simulink model "lab_single_phse_inv"  (R2020a)
settings: Solver=VariableStepAuto  StartTime=0.0  StopTime=0.1  RelTol=1e-3
libraries: powerlib x9, simulink x1
settings Model: Creator=Manish  LastModifiedBy=Manish
settings DataIOCC: ReturnWorkspaceOutputs=off

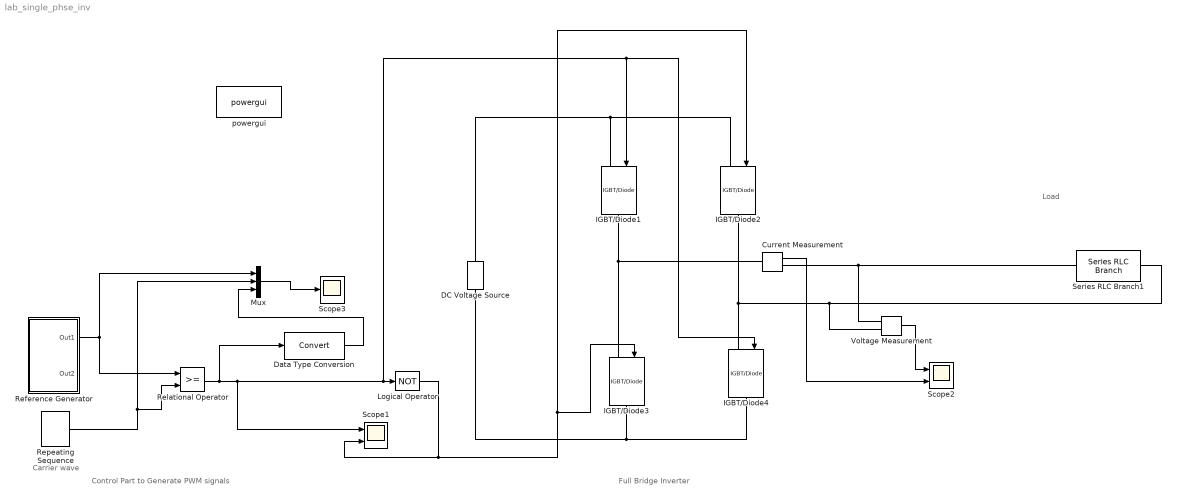
== system lab_single_phse_inv ==
  note: Full Bridge Inverter
  note: Load
  note: Control Part to
      | Generate PWM signals
  note: Carrier wave
  Current Measurement : powerlib/Measurements/Current Measurement  PhasorSimulation=off  OutputType=Complex  PSBequivalent=0
  DC Voltage Source : powerlib/Electrical Sources/DC Voltage Source  Amplitude=15  Measurements=None
  Data Type Conversion : DataTypeConversion
  IGBT/Diode{1..4} (4 alike) : powerlib/Power Electronics/IGBT//Diode  Ron=1e-3  Rs=1e5  Cs=inf  Measurements=off
  Logical Operator : Logic  Operator=NOT  AllPortsSameDT=off  OutDataTypeStr=boolean
  Mux : Mux  Inputs=3
  Reference Generator : Subsystem
  Relational Operator : RelationalOperator  RndMeth=Nearest
  Repeating Sequence : simulink/Sources/Repeating Sequence  rep_seq_t=[0 0.25 0.5 0.75 1]/1000  rep_seq_y=[0 1 0 -1 0]
  Scope1 : Scope  NumInputPorts=2
  Scope2 : Scope  NumInputPorts=2
  Scope3 : Scope
  Series RLC Branch1 : powerlib/Elements/Series RLC Branch  LConnTagsString=__new0  RConnTagsString=__new0  BranchType=RL  Resistance=10  Inductance=10e-3  SetiL0=off  InitialCurrent=0  Capacitance=1e-6  Setx0=off  InitialVoltage=0  Measurements=None
  Voltage Measurement : powerlib/Measurements/Voltage Measurement  PhasorSimulation=off  OutputType=Complex  PSBequivalent=0
  powergui : powerlib/powergui  Priority=1  SimulationMode=Discrete  SampleTime=1e-6  frequency=60  Iterations=50  frequencyindice=0  Pbase=100e6  ErrMax=1e-4  UnitsV=kV  UnitsW=MW  buscounter=0  FunctionMessages=off  echomessages=off  EnableUseOfTLC=off  CurrentSourceSwitches=off  DisableSnubberDevices=off  DisableRonSwitches=off  DisableVfSwitches=off  DisplayEquations=off  AutomaticDiscreteSolvers=off  SolverType=Tustin/Backward Euler (TBE)  Interpol=off  ExternalGateDelay=off  methode=off  Ts=100  x0status=blocks  SPID=on  SwTol=0  HookPort=off  NonlinearTolerance=1e-4  nMaxIteration=100  ContinueOnMaxIteration=off  RestoreLinks=warning  ResistiveCurrentMeasurement=off  Frange=[0:2:500]  Ylog=off  Xlog=on  ShowGrid=off  save=off  variable=ZData  structure=voltage_current  ZoomFFT=off  StartTime=0  cycles=1  DisplayStyle=2  fundamental=50  FreqAxis=off  MaxFrequency=10000  frequencyindicesteady=1  RmsSteady=1  display=off
  wires:
  Reference Generator/1(Out1) -> Relational Operator/1, Mux/1
  Repeating Sequence/1 -> Mux/2, Relational Operator/2
  Relational Operator/1 -> Data Type Conversion/1, IGBT/Diode4/1, IGBT/Diode1/1, Logical Operator/1, Scope1/1
  Logical Operator/1 -> IGBT/Diode3/1, IGBT/Diode2/1, Scope1/2
  Voltage Measurement/1 -> Scope2/1
  Current Measurement/1 -> Scope2/2
  Mux/1 -> Scope3/1
  Data Type Conversion/1 -> Mux/3
  connections:
  DC Voltage Source/RConn1 -- IGBT/Diode2/LConn1 -- IGBT/Diode1/LConn1
  DC Voltage Source/LConn1 -- IGBT/Diode4/RConn1 -- IGBT/Diode3/RConn1
  Current Measurement/LConn1 -- IGBT/Diode3/LConn1 -- IGBT/Diode1/RConn1
  Voltage Measurement/LConn1 -- Series RLC Branch1/LConn1 -- Current Measurement/RConn1
  Voltage Measurement/LConn2 -- Series RLC Branch1/RConn1 -- IGBT/Diode2/RConn1 -- IGBT/Diode4/LConn1

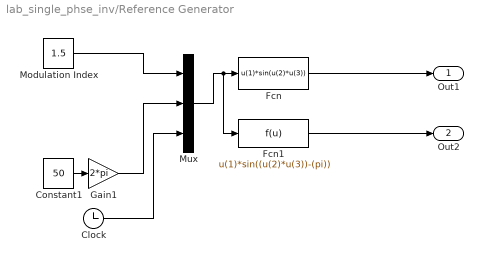
== system lab_single_phse_inv/Reference Generator ==
  Clock : Clock
      settings: Decimation=100
  Constant1 : Constant  Value=50
  Fcn : Fcn  Expr=u(1)*sin(u(2)*u(3))
  Fcn1 : Fcn  Expr=u(1)*sin((u(2)*u(3))-(pi))
  Gain1 : Gain  Gain=2*pi
  Modulation Index : Constant  Value=1.5
  Mux : Mux  Inputs=3
  Out1 : Outport
  Out2 : Outport  Port=2
  wires:
  Gain1/1 -> Mux/2
  Mux/1 -> Fcn/1, Fcn1/1
  Fcn/1 -> Out1/1
  Fcn1/1 -> Out2/1
  Modulation Index/1 -> Mux/1
  Clock/1 -> Mux/3
  Constant1/1 -> Gain1/1
